simulink model "Avoiding_Obstacle"  (R2015b)
settings: Solver=VariableStepAuto  StartTime=0.0  StopTime=inf  RelTol=1e-3
values from neighbouring files (symbols this model uses):
  waypoints = getWaypoints()    [start.m]
undefined symbols (not defined in the file or in its folder): Angular, Linear
libraries: robotlib x4
settings Model: Creator=exbot  LastModifiedBy=exbot

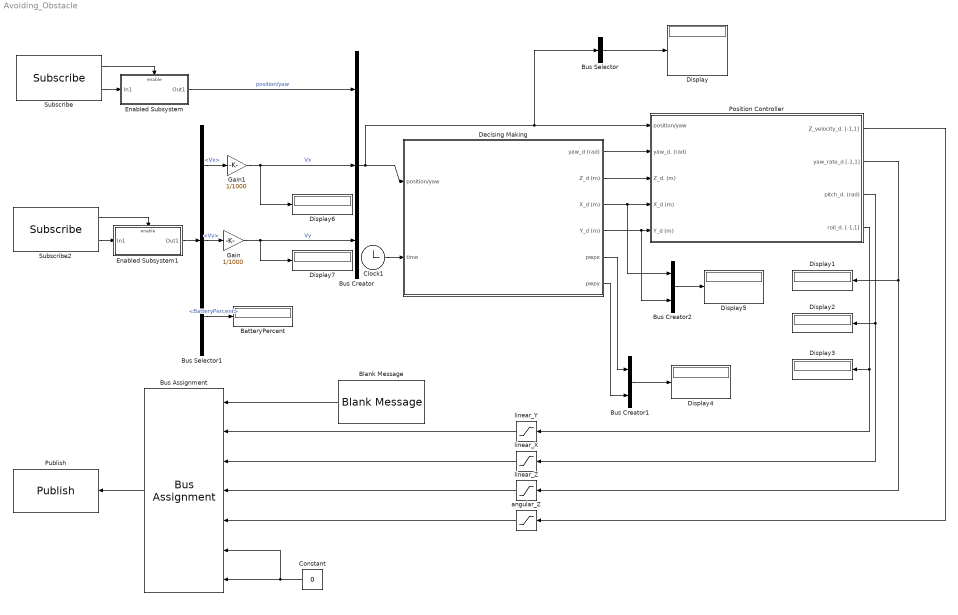
== system Avoiding_Obstacle ==
  BatteryPercent : Display
  Blank Message : robotlib/Blank Message  SourceLibraryInfo=This block requires Robotics System Toolbox  messageType=geometry_msgs/Twist  SampleTime=inf
  Bus Assignment : BusAssignment  AssignedSignals=Linear.Y,Linear.X,Angular.Z,Linear.Z,Angular.X,Angular.Y
  Bus Creator : BusCreator  Inputs=3
  Bus Creator1 : BusCreator  Inputs=2
  Bus Creator2 : BusCreator  Inputs=2
  Bus Selector : BusSelector  OutputSignals=position/yaw.XE,position/yaw.YE,position/yaw.YawE  OutputAsBus=on
  Bus Selector1 : BusSelector  OutputSignals=Vx,Vy,BatteryPercent
  Clock1 : Clock
  Constant : Constant  Value=0
  Decising Making : Subsystem
  Display{,1..7} (8 alike) : Display
  Enabled Subsystem : Subsystem  TreatAsAtomicUnit=on
  Enabled Subsystem1 : Subsystem  TreatAsAtomicUnit=on
  Gain : Gain  Gain=1/1000
  Gain1 : Gain  Gain=1/1000
  Position Controller : Subsystem  AncestorBlock=ARBlocks/Baseline Controller
  Publish : robotlib/Publish  SourceLibraryInfo=This block requires Robotics System Toolbox  topicSource=Select from ROS network  topic=/cmd_vel  messageType=geometry_msgs/Twist  messageQueueLength=1
  Subscribe : robotlib/Subscribe  SourceLibraryInfo=This block requires Robotics System Toolbox  topicSource=Select from ROS network  topic=/vpsnavdata  messageType=vps_driver/vps_navdata  sampleTime=-1  messageQueueLength=1
  Subscribe2 : robotlib/Subscribe  SourceLibraryInfo=This block requires Robotics System Toolbox  topicSource=Select from ROS network  topic=/ardrone/navdata  messageType=ardrone_autonomy/Navdata  sampleTime=-1  messageQueueLength=1
  angular_Z : Saturate  UpperLimit=0.1  LowerLimit=-0.1
  linear_X : Saturate  UpperLimit=0.1  LowerLimit=-0.1
  linear_Y : Saturate  UpperLimit=0.1  LowerLimit=-0.1
  linear_Z : Saturate  UpperLimit=0.1  LowerLimit=-0.1
  wires:
  Decising Making/3(X_d (m)) -> Bus Creator2/1, Position Controller/4(X_d (m))
  Decising Making/4(Y_d (m)) -> Bus Creator2/2, Position Controller/5(Y_d (m))
  Decising Making/2(Z_d (m)) -> Position Controller/3(Z_d. (m))
  Clock1/1 -> Decising Making/2(time)
  Decising Making/1(yaw_d (rad)) -> Position Controller/2(yaw_d. (rad))
  Bus Selector1/2 -> Gain/1  "<Vy>"
  Gain/1 -> Bus Creator/3, Display7/1  "Vy"
  Bus Selector1/1 -> Gain1/1  "<Vx>"
  Bus Creator/1 -> Decising Making/1(position/yaw), Bus Selector/1, Position Controller/1(" position/yaw ")
  Enabled Subsystem/1(Out1) -> Bus Creator/1  "position/yaw"
  Enabled Subsystem1/1(Out1) -> Bus Selector1/1
  Bus Selector1/3 -> BatteryPercent/1  "<BatteryPercent>"
  Blank Message/1 -> Bus Assignment/1
  Position Controller/1(Z_velocity_d. [-1,1]) -> angular_Z/1
  Position Controller/2(yaw_rate_d [-1,1]) -> Display1/1, linear_Z/1
  Position Controller/3(pitch_d. (rad)) -> linear_X/1, Display2/1
  Position Controller/4(roll_d. [-1,1]) -> linear_Y/1, Display3/1
  Bus Assignment/1 -> Publish/1
  Subscribe/2 -> Enabled Subsystem/1(In1)
  Subscribe/1 -> Enabled Subsystem/Enable
  Subscribe2/2 -> Enabled Subsystem1/1(In1)
  Subscribe2/1 -> Enabled Subsystem1/Enable
  Constant/1 -> Bus Assignment/6, Bus Assignment/7
  linear_Y/1 -> Bus Assignment/2
  angular_Z/1 -> Bus Assignment/5
  linear_Z/1 -> Bus Assignment/4
  linear_X/1 -> Bus Assignment/3
  Gain1/1 -> Bus Creator/2, Display6/1  "Vx"
  Bus Selector/1 -> Display/1
  Decising Making/5(pwpx) -> Bus Creator1/1
  Decising Making/6(pwpy) -> Bus Creator1/2
  Bus Creator1/1 -> Display4/1
  Bus Creator2/1 -> Display5/1

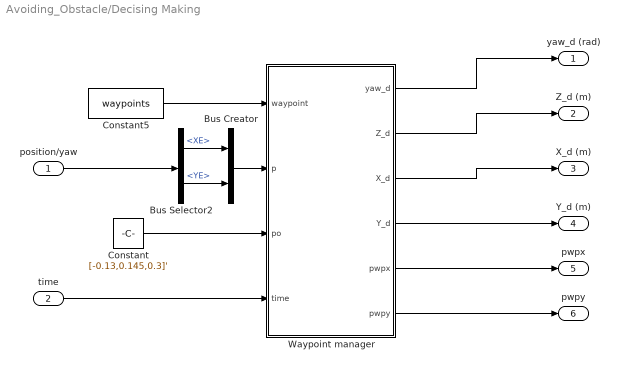
== system Avoiding_Obstacle/Decising Making ==
  position/yaw : Inport
  time : Inport  Port=2
  Bus Creator : BusCreator  Inputs=2
  Bus Selector2 : BusSelector  OutputSignals=position/yaw.XE,position/yaw.YE
  Constant : Constant  Value=[-0.13,0.145,0.3]'
  Constant5 : Constant  Value=waypoints  VectorParams1D=off
  "Waypoint manager " : MATLAB Function  TreatAsAtomicUnit=on
  yaw_d (rad) : Outport
  Z_d (m) : Outport  Port=2
  X_d (m) : Outport  Port=3
  Y_d (m) : Outport  Port=4
  pwpx : Outport  Port=5
  pwpy : Outport  Port=6
  wires:
  position/yaw/1 -> Bus Selector2/1
  "Waypoint manager "/2(Z_d) -> Z_d (m)/1
  "Waypoint manager "/3(X_d) -> X_d (m)/1
  "Waypoint manager "/4(Y_d) -> Y_d (m)/1
  time/1 -> "Waypoint manager "/4(time)
  "Waypoint manager "/5(pwpx) -> pwpx/1
  "Waypoint manager "/1(yaw_d) -> yaw_d (rad)/1
  Constant5/1 -> "Waypoint manager "/1(waypoint)
  Bus Selector2/1 -> Bus Creator/1  "<XE>"
  Bus Selector2/2 -> Bus Creator/2  "<YE>"
  Bus Creator/1 -> "Waypoint manager "/2(p)
  Constant/1 -> "Waypoint manager "/3(po)
  "Waypoint manager "/6(pwpy) -> pwpy/1

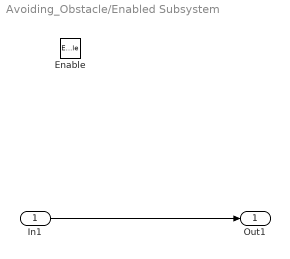
== system Avoiding_Obstacle/Enabled Subsystem ==
  In1 : Inport
  Enable : EnablePort
  Out1 : Outport
  wires:
  In1/1 -> Out1/1

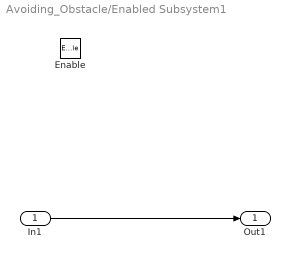
== system Avoiding_Obstacle/Enabled Subsystem1 ==
  In1 : Inport
  Enable : EnablePort
  Out1 : Outport
  wires:
  In1/1 -> Out1/1

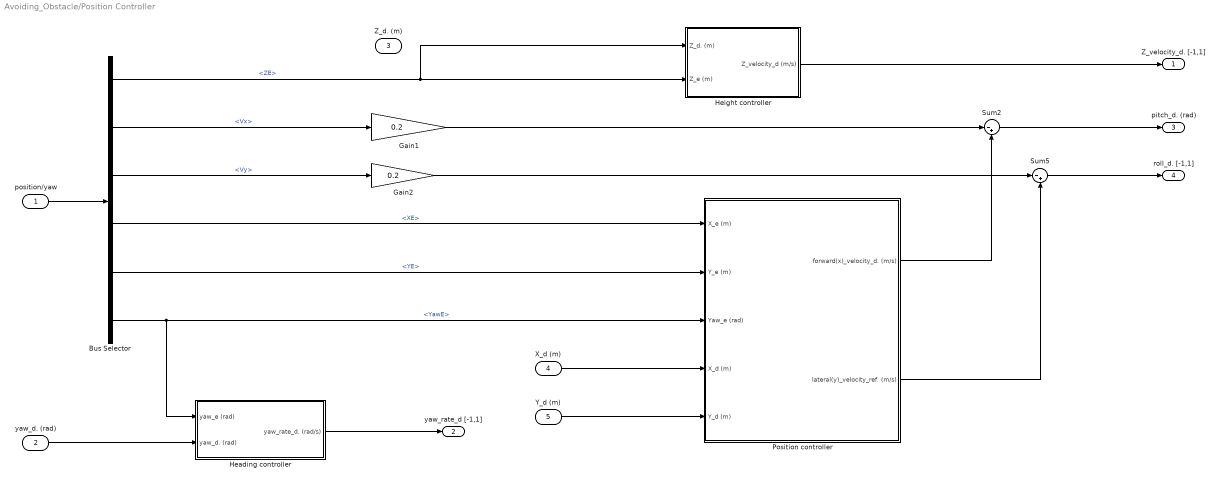
== system Avoiding_Obstacle/Position Controller ==
  " position/yaw " : Inport
  yaw_d. (rad) : Inport  Port=2
  Z_d. (m) : Inport  Port=3
  X_d (m) : Inport  Port=4
  Y_d (m) : Inport  Port=5
  Bus Selector : BusSelector  OutputSignals=position/yaw.ZE,Vx,Vy,position/yaw.XE,position/yaw.YE,position/yaw.YawE
  Gain1 : Gain  Gain=0.2
  Gain2 : Gain  Gain=0.2
  Heading controller : Subsystem
  "Height controller " : Subsystem
  Position controller : Subsystem
  Sum2 : Sum  Inputs=|-+
  Sum5 : Sum  Inputs=|-+
  Z_velocity_d. [-1,1] : Outport
  yaw_rate_d [-1,1] : Outport  Port=2
  pitch_d. (rad) : Outport  Port=3
  roll_d. [-1,1] : Outport  Port=4
  wires:
  Position controller/2(lateral(y)_velocity_ref. (m/s)) -> Sum5/2
  Gain2/1 -> Sum5/1
  Bus Selector/3 -> Gain2/1  "<Vy>"
  Position controller/1(forward(x)_velocity_d. (m/s)) -> Sum2/2
  Gain1/1 -> Sum2/1
  Bus Selector/6 -> Position controller/3(Yaw_e (rad)), Heading controller/1(yaw_e (rad))  "<YawE>"
  " position/yaw "/1 -> Bus Selector/1
  Bus Selector/1 -> "Height controller "/1(Z_d. (m)), "Height controller "/2(Z_e (m))  "<ZE>"
  "Height controller "/1(Z_velocity_d (m/s)) -> Z_velocity_d. [-1,1]/1
  Bus Selector/2 -> Gain1/1  "<Vx>"
  Heading controller/1(yaw_rate_d. (rad/s)) -> yaw_rate_d [-1,1]/1
  Bus Selector/4 -> Position controller/1(X_e (m))  "<XE>"
  Bus Selector/5 -> Position controller/2(Y_e (m))  "<YE>"
  X_d (m)/1 -> Position controller/4(X_d (m))
  Y_d (m)/1 -> Position controller/5(Y_d (m))
  Sum2/1 -> pitch_d. (rad)/1
  Sum5/1 -> roll_d. [-1,1]/1
  yaw_d. (rad)/1 -> Heading controller/2(yaw_d. (rad))

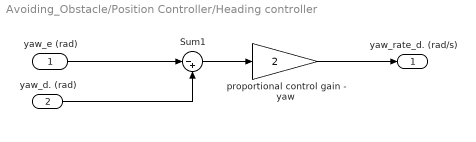
== system Avoiding_Obstacle/Position Controller/Heading controller ==
  yaw_e (rad) : Inport
  yaw_d. (rad) : Inport  Port=2
  Sum1 : Sum  Inputs=|-+
  proportional control gain - yaw : Gain  Gain=2
  yaw_rate_d. (rad/s) : Outport
  wires:
  Sum1/1 -> proportional control gain - yaw/1
  proportional control gain - yaw/1 -> yaw_rate_d. (rad/s)/1
  yaw_e (rad)/1 -> Sum1/1
  yaw_d. (rad)/1 -> Sum1/2

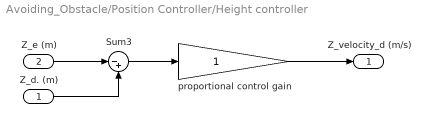
== system Avoiding_Obstacle/Position Controller/Height controller  ==
  Z_d. (m) : Inport
  Z_e (m) : Inport  Port=2
  Sum3 : Sum  Inputs=|-+
  proportional control gain : Gain
  Z_velocity_d (m/s) : Outport
  wires:
  proportional control gain/1 -> Z_velocity_d (m/s)/1
  Sum3/1 -> proportional control gain/1
  Z_e (m)/1 -> Sum3/1
  Z_d. (m)/1 -> Sum3/2

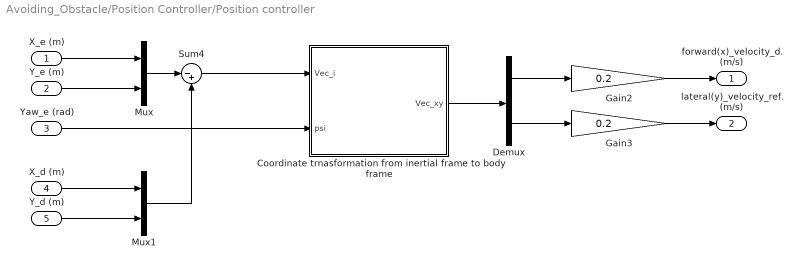
== system Avoiding_Obstacle/Position Controller/Position controller ==
  X_e (m) : Inport
  Y_e (m) : Inport  Port=2
  Yaw_e (rad) : Inport  Port=3
  X_d (m) : Inport  Port=4
  Y_d (m) : Inport  Port=5
  "Coordinate trnasformation from inertial frame to body frame " : MATLAB Function  TreatAsAtomicUnit=on
  Demux : Demux  Outputs=2
  Gain2 : Gain  Gain=0.2
  Gain3 : Gain  Gain=0.2
  Mux : Mux  Inputs=2
  Mux1 : Mux  Inputs=2
  Sum4 : Sum  Inputs=|-+
  forward(x)_velocity_d. (m/s) : Outport
  lateral(y)_velocity_ref. (m/s) : Outport  Port=2
  wires:
  Gain2/1 -> forward(x)_velocity_d. (m/s)/1
  Yaw_e (rad)/1 -> "Coordinate trnasformation from inertial frame to body frame "/2(psi)
  "Coordinate trnasformation from inertial frame to body frame "/1(Vec_xy) -> Demux/1
  Mux1/1 -> Sum4/2
  Sum4/1 -> "Coordinate trnasformation from inertial frame to body frame "/1(Vec_i)
  Y_e (m)/1 -> Mux/2
  X_e (m)/1 -> Mux/1
  Mux/1 -> Sum4/1
  X_d (m)/1 -> Mux1/1
  Y_d (m)/1 -> Mux1/2
  Demux/1 -> Gain2/1
  Demux/2 -> Gain3/1
  Gain3/1 -> lateral(y)_velocity_ref. (m/s)/1

== matlab function Avoiding_Obstacle/Position Controller/Position controller/Coordinate trnasformation from inertial frame to body frame  ==
  data: Vec_i input; Vec_xy output; psi input
function Vec_xy  = fcn(Vec_i , psi)
%#codegen
T = [cos(psi) sin(psi) ; -sin(psi) cos(psi)] ; 
Vec_xy = T*Vec_i(1:2,1);

== matlab function Avoiding_Obstacle/Decising Making/Waypoint manager  ==
  data: yaw_d output; Z_d output; waypoint input; p input; po input; X_d output; Y_d output; time input; pwpx output; pwpy output
function [yaw_d, Z_d,  X_d, Y_d, pwpx,pwpy]       = fcn(waypoint, p, po,time )

nPoints = size(waypoint, 2) ;
persistent wpointer;
persistent t0 ;
persistent pd;

if isempty(wpointer)
    wpointer = 1;
end

if isempty(t0)
    t0 = 0;
end

if isempty(pd)
    pd = [0 0]';
end


if ( norm(p - waypoint(1:2, wpointer) )< 0.3 )    
    if(wpointer ~= nPoints)        
        if (t0 ==0)
            t0 = time;
        else
            if (time - t0 > waypoint(5, wpointer))               
                 if(wpointer < nPoints)
                    wpointer = wpointer+ 1;
                    t0 = 0;
                 end                
            end
        end         
    end    
end

pd = p + 1*satgd(waypoint(1:2,wpointer) - p,1.5)...
          -0.15*[0 -1;1 0]*(po(1:2)-p)/(((p-po(1:2))'*(p-po(1:2))-po(3)^2)^2);



%% Outputs
Z_d =  waypoint(3, wpointer) ;
yaw_d = waypoint(4, wpointer) ;
X_d = pd(1) ;
Y_d = pd(2) ;
pwpx = waypoint(1, wpointer) ;
pwpy = waypoint(2, wpointer) ;
